simulink model "problem3"  (R2020b)
settings: Solver=ode45  StartTime=0.0  StopTime=120  RelTol=1e-3
values from neighbouring files (symbols this model uses):
  b = 2.0    [problem3datadic.sldd]
  m = 10.0    [problem3datadic.sldd]
settings Model: Creator=Nitin  LastModifiedBy=Nitin

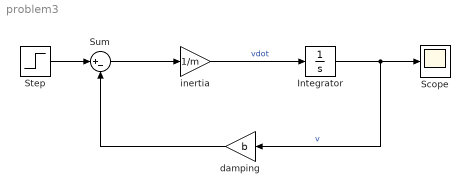
== system problem3 ==
  Integrator : Integrator
  Scope : Scope
  Step : Step  Time=0  After=u  SampleTime=0
  Sum : Sum  Inputs=|+-
  damping : Gain  Gain=b
  inertia : Gain  Gain=1/m
  wires:
  inertia/1 -> Integrator/1  "vdot"
  Integrator/1 -> Scope/1, damping/1  "v"
  Sum/1 -> inertia/1
  damping/1 -> Sum/2
  Step/1 -> Sum/1
